simulink model "simulink_model"  (R2023b)
settings: Solver=VariableStepAuto  StartTime=0.0  StopTime=0.0005  RelTol=1e-3
values from neighbouring files (symbols this model uses):
  A = [0 1/C;-1/L -R/L]    [values_rlc.m]
  B = [0;1/L]    [values_rlc.m]
settings Model: Creator=jacei  LastModifiedBy=jacei

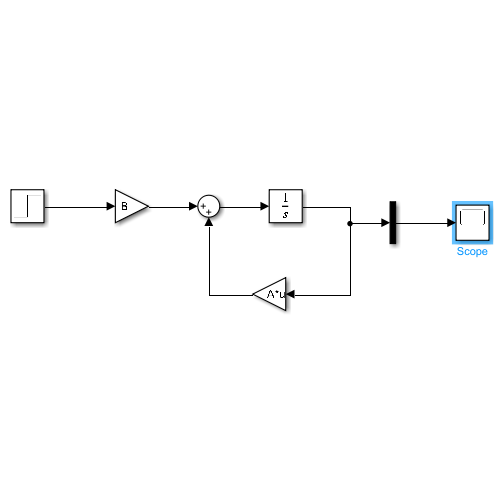
[thumbnail: Simulink's stored preview of the top-level diagram]
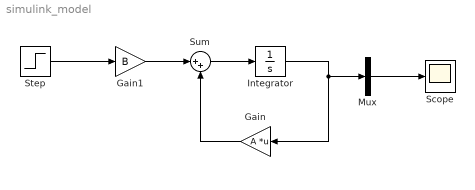
== system simulink_model ==
  Gain : Gain  Gain=A  Multiplication=Matrix(K*u)
  Gain1 : Gain  Gain=B
  Integrator : Integrator
  Mux : Mux  Inputs=1
  Scope : Scope
  Step : Step  Time=2  Before=12  After=12  SampleTime=0
  Sum : Sum  Inputs=|++
  wires:
  Gain1/1 -> Sum/1
  Sum/1 -> Integrator/1
  Gain/1 -> Sum/2
  Step/1 -> Gain1/1
  Integrator/1 -> Mux/1, Gain/1
  Mux/1 -> Scope/1
